simulink model "fifteenbands"  (R2021b)
settings: Solver=VariableStepAuto  StartTime=0.0  StopTime=inf  RelTol=1e-3
values from neighbouring files (symbols this model uses):
  C = {name "-" "-" "-" "-" "-" "-" "-" "-" "-" gain10 gain11 gain12}    [Equalizer.m]
libraries: dspfdesign x13, dspmathops x12, dspsnks4 x1, dspvision x1
settings Model: PacingRate=100  Creator=DSP  LastModifiedBy=DSP

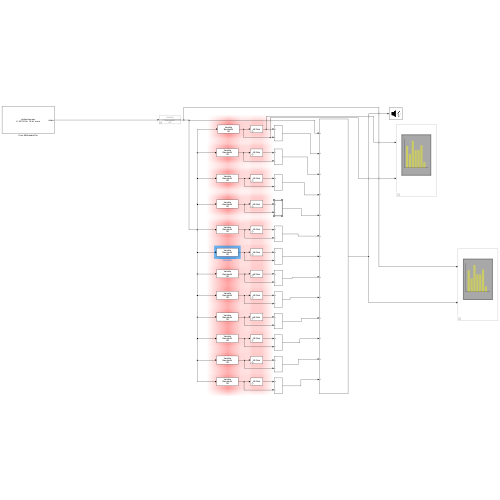
[thumbnail: Simulink's stored preview of the top-level diagram]
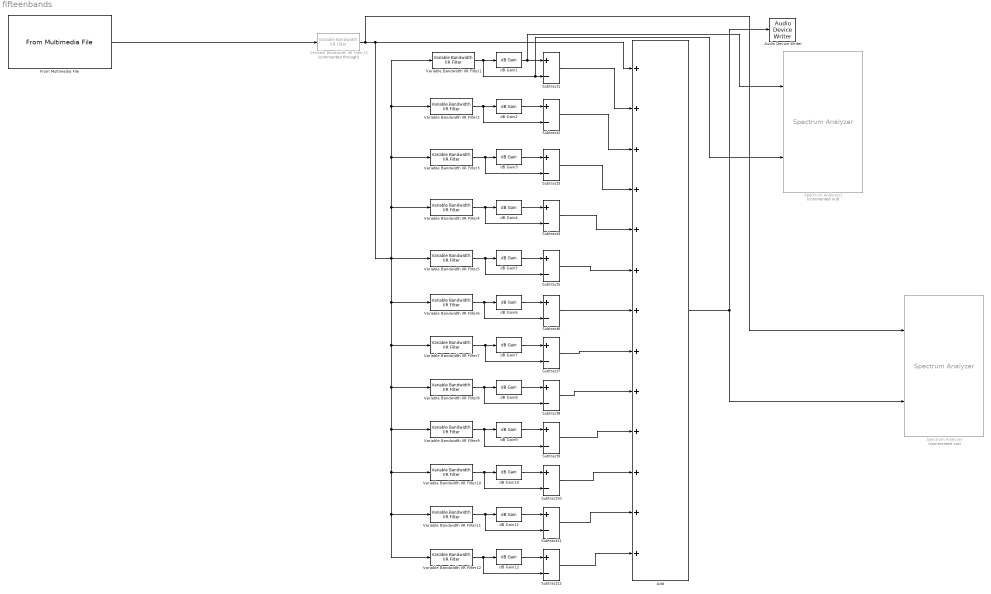
== system fifteenbands ==
  Add : Sum  Inputs=+++++++++++++
  Audio Device Writer : dspsnks4/Audio Device Writer  Driver=DirectSound  Device=Default  InheritSampleRate=on  SampleRate=44100  BitDepth=16-bit integer  BufferSize=4096  NumBuffers=10  DefaultOutputChannelMapping=on  OutputChannelMapping=1:2  OutputNumUnderrunSamples=off  DriverIdx=1  DeviceWarnFlag=''
  From Multimedia File : dspvision/From Multimedia File  inputFilename=C:\Users\DSP\Desktop\Equalizer\SongFolder\whitenoise.wav  readRange=[1 Inf]  loop=on  numPlays=inf  outputStreams=Audio only  videoDataType=single  audioDataType=double  inheritSampleTime=on  userDefinedSampleTime=1/30  noAudioOutput=off  isIntensityVideo=off  fourcc=RGB  colorVideoFormat=Separate color signals  outputEOF=off  dataOrg=Column-major  audioFrameSize=1024  computeAudioFrameSize=off  outSamplingMode=Sample based
  Spectrum Analyzer : SpectrumAnalyzer  Commented=on  NumInputPorts=2
  Spectrum Analyzer1 : SpectrumAnalyzer  Commented=on  NumInputPorts=2
  Subtract{1..12} (12 alike) : Sum  Inputs=+-
  Variable Bandwidth IIR Filter1 : dspfdesign/Variable Bandwidth IIR Filter  FilterType=Bandpass  FilterOrder=4  PassbandFrequencyPort=off  PassbandFrequency=512  CenterFrequencyPort=off  CenterFrequency=freq1  BandwidthPort=off  Bandwidth=bw1  PassbandRipple=1  StopbandAttenuation=60  InheritSampleRate=off  SampleRate=44100  SimulateUsing=Code generation
      settings: SourceProductBaseCode=DS
  Variable Bandwidth IIR Filter10 : dspfdesign/Variable Bandwidth IIR Filter  FilterType=Bandpass  FilterOrder=4  PassbandFrequencyPort=off  PassbandFrequency=512  CenterFrequencyPort=off  CenterFrequency=freq10  BandwidthPort=off  Bandwidth=bw10  PassbandRipple=1  StopbandAttenuation=60  InheritSampleRate=off  SampleRate=44100  SimulateUsing=Code generation
      settings: SourceProductBaseCode=DS
  Variable Bandwidth IIR Filter11 : dspfdesign/Variable Bandwidth IIR Filter  FilterType=Bandpass  FilterOrder=4  PassbandFrequencyPort=off  PassbandFrequency=512  CenterFrequencyPort=off  CenterFrequency=freq11  BandwidthPort=off  Bandwidth=bw11  PassbandRipple=1  StopbandAttenuation=60  InheritSampleRate=off  SampleRate=44100  SimulateUsing=Code generation
      settings: SourceProductBaseCode=DS
  Variable Bandwidth IIR Filter12 : dspfdesign/Variable Bandwidth IIR Filter  FilterType=Bandpass  FilterOrder=4  PassbandFrequencyPort=off  PassbandFrequency=512  CenterFrequencyPort=off  CenterFrequency=freq12  BandwidthPort=off  Bandwidth=bw12  PassbandRipple=1  StopbandAttenuation=60  InheritSampleRate=off  SampleRate=44100  SimulateUsing=Code generation
      settings: SourceProductBaseCode=DS
  Variable Bandwidth IIR Filter13 : dspfdesign/Variable Bandwidth IIR Filter  Commented=through  FilterType=Lowpass  FilterOrder=4  PassbandFrequencyPort=off  PassbandFrequency=2000  CenterFrequencyPort=off  CenterFrequency=44100/4  BandwidthPort=off  Bandwidth=7680  PassbandRipple=1  StopbandAttenuation=60  InheritSampleRate=off  SampleRate=44100  SimulateUsing=Code generation
      settings: SourceProductBaseCode=DS
  Variable Bandwidth IIR Filter2 : dspfdesign/Variable Bandwidth IIR Filter  FilterType=Bandpass  FilterOrder=4  PassbandFrequencyPort=off  PassbandFrequency=512  CenterFrequencyPort=off  CenterFrequency=freq2  BandwidthPort=off  Bandwidth=bw2  PassbandRipple=1  StopbandAttenuation=60  InheritSampleRate=off  SampleRate=44100  SimulateUsing=Code generation
      settings: SourceProductBaseCode=DS
  Variable Bandwidth IIR Filter3 : dspfdesign/Variable Bandwidth IIR Filter  FilterType=Bandpass  FilterOrder=4  PassbandFrequencyPort=off  PassbandFrequency=512  CenterFrequencyPort=off  CenterFrequency=freq3  BandwidthPort=off  Bandwidth=bw3  PassbandRipple=1  StopbandAttenuation=60  InheritSampleRate=off  SampleRate=44100  SimulateUsing=Code generation
      settings: SourceProductBaseCode=DS
  Variable Bandwidth IIR Filter4 : dspfdesign/Variable Bandwidth IIR Filter  FilterType=Bandpass  FilterOrder=4  PassbandFrequencyPort=off  PassbandFrequency=512  CenterFrequencyPort=off  CenterFrequency=freq4  BandwidthPort=off  Bandwidth=bw4  PassbandRipple=1  StopbandAttenuation=60  InheritSampleRate=off  SampleRate=44100  SimulateUsing=Code generation
      settings: SourceProductBaseCode=DS
  Variable Bandwidth IIR Filter5 : dspfdesign/Variable Bandwidth IIR Filter  FilterType=Bandpass  FilterOrder=4  PassbandFrequencyPort=off  PassbandFrequency=512  CenterFrequencyPort=off  CenterFrequency=freq5  BandwidthPort=off  Bandwidth=bw5  PassbandRipple=1  StopbandAttenuation=60  InheritSampleRate=off  SampleRate=44100  SimulateUsing=Code generation
      settings: SourceProductBaseCode=DS
  Variable Bandwidth IIR Filter6 : dspfdesign/Variable Bandwidth IIR Filter  FilterType=Bandpass  FilterOrder=4  PassbandFrequencyPort=off  PassbandFrequency=512  CenterFrequencyPort=off  CenterFrequency=freq6  BandwidthPort=off  Bandwidth=bw6  PassbandRipple=1  StopbandAttenuation=60  InheritSampleRate=off  SampleRate=44100  SimulateUsing=Code generation
      settings: SourceProductBaseCode=DS
  Variable Bandwidth IIR Filter7 : dspfdesign/Variable Bandwidth IIR Filter  FilterType=Bandpass  FilterOrder=4  PassbandFrequencyPort=off  PassbandFrequency=512  CenterFrequencyPort=off  CenterFrequency=freq7  BandwidthPort=off  Bandwidth=bw7  PassbandRipple=1  StopbandAttenuation=60  InheritSampleRate=off  SampleRate=44100  SimulateUsing=Code generation
      settings: SourceProductBaseCode=DS
  Variable Bandwidth IIR Filter8 : dspfdesign/Variable Bandwidth IIR Filter  FilterType=Bandpass  FilterOrder=4  PassbandFrequencyPort=off  PassbandFrequency=512  CenterFrequencyPort=off  CenterFrequency=freq8  BandwidthPort=off  Bandwidth=bw8  PassbandRipple=1  StopbandAttenuation=60  InheritSampleRate=off  SampleRate=44100  SimulateUsing=Code generation
      settings: SourceProductBaseCode=DS
  Variable Bandwidth IIR Filter9 : dspfdesign/Variable Bandwidth IIR Filter  FilterType=Bandpass  FilterOrder=4  PassbandFrequencyPort=off  PassbandFrequency=512  CenterFrequencyPort=off  CenterFrequency=freq9  BandwidthPort=off  Bandwidth=bw9  PassbandRipple=1  StopbandAttenuation=60  InheritSampleRate=off  SampleRate=44100  SimulateUsing=Code generation
      settings: SourceProductBaseCode=DS
  dB Gain1 : dspmathops/dB Gain  dB=gain1  intype=Amplitude
      settings: SourceProductBaseCode=DS
  dB Gain10 : dspmathops/dB Gain  dB=gain10  intype=Amplitude
      settings: SourceProductBaseCode=DS
  dB Gain11 : dspmathops/dB Gain  dB=gain11  intype=Amplitude
      settings: SourceProductBaseCode=DS
  dB Gain12 : dspmathops/dB Gain  dB=gain12  intype=Amplitude
      settings: SourceProductBaseCode=DS
  dB Gain2 : dspmathops/dB Gain  dB=gain2  intype=Amplitude
      settings: SourceProductBaseCode=DS
  dB Gain3 : dspmathops/dB Gain  dB=gain3  intype=Amplitude
      settings: SourceProductBaseCode=DS
  dB Gain4 : dspmathops/dB Gain  dB=gain4  intype=Amplitude
      settings: SourceProductBaseCode=DS
  dB Gain5 : dspmathops/dB Gain  dB=gain5  intype=Amplitude
      settings: SourceProductBaseCode=DS
  dB Gain6 : dspmathops/dB Gain  dB=gain6  intype=Amplitude
      settings: SourceProductBaseCode=DS
  dB Gain7 : dspmathops/dB Gain  dB=gain7  intype=Amplitude
      settings: SourceProductBaseCode=DS
  dB Gain8 : dspmathops/dB Gain  dB=gain8  intype=Amplitude
      settings: SourceProductBaseCode=DS
  dB Gain9 : dspmathops/dB Gain  dB=gain9  intype=Amplitude
      settings: SourceProductBaseCode=DS
  wires:
  Variable Bandwidth IIR Filter1/1 -> Spectrum Analyzer1/2, Subtract1/2, dB Gain1/1
  Variable Bandwidth IIR Filter2/1 -> Subtract2/2, dB Gain2/1
  Variable Bandwidth IIR Filter3/1 -> Subtract3/2, dB Gain3/1
  dB Gain1/1 -> Spectrum Analyzer1/1, Subtract1/1
  Subtract1/1 -> Add/2
  dB Gain2/1 -> Subtract2/1
  dB Gain3/1 -> Subtract3/1
  Subtract2/1 -> Add/3
  Subtract3/1 -> Add/4
  Variable Bandwidth IIR Filter4/1 -> Subtract4/2, dB Gain4/1
  Variable Bandwidth IIR Filter5/1 -> Subtract5/2, dB Gain5/1
  dB Gain4/1 -> Subtract4/1
  dB Gain5/1 -> Subtract5/1
  Subtract4/1 -> Add/5
  Subtract5/1 -> Add/6
  Variable Bandwidth IIR Filter6/1 -> Subtract6/2, dB Gain6/1
  Variable Bandwidth IIR Filter7/1 -> Subtract7/2, dB Gain7/1
  Variable Bandwidth IIR Filter8/1 -> Subtract8/2, dB Gain8/1
  dB Gain6/1 -> Subtract6/1
  dB Gain7/1 -> Subtract7/1
  dB Gain8/1 -> Subtract8/1
  dB Gain9/1 -> Subtract9/1
  Variable Bandwidth IIR Filter9/1 -> Subtract9/2, dB Gain9/1
  dB Gain10/1 -> Subtract10/1
  Variable Bandwidth IIR Filter10/1 -> Subtract10/2, dB Gain10/1
  dB Gain11/1 -> Subtract11/1
  Variable Bandwidth IIR Filter11/1 -> Subtract11/2, dB Gain11/1
  Variable Bandwidth IIR Filter12/1 -> Subtract12/2, dB Gain12/1
  dB Gain12/1 -> Subtract12/1
  Subtract6/1 -> Add/7
  Subtract7/1 -> Add/8
  Subtract8/1 -> Add/9
  Subtract9/1 -> Add/10
  Subtract10/1 -> Add/11
  Subtract11/1 -> Add/12
  Subtract12/1 -> Add/13
  Variable Bandwidth IIR Filter13/1 -> Spectrum Analyzer/1, Add/1, Variable Bandwidth IIR Filter1/1, Variable Bandwidth IIR Filter2/1, Variable Bandwidth IIR Filter3/1, Variable Bandwidth IIR Filter4/1, Variable Bandwidth IIR Filter12/1, Variable Bandwidth IIR Filter11/1, Variable Bandwidth IIR Filter10/1, Variable Bandwidth IIR Filter9/1, Variable Bandwidth IIR Filter8/1, Variable Bandwidth IIR Filter7/1, Variable Bandwidth IIR Filter6/1, Variable Bandwidth IIR Filter5/1
  Add/1 -> Audio Device Writer/1, Spectrum Analyzer/2
  From Multimedia File/1 -> Variable Bandwidth IIR Filter13/1
